simulink model "simulate_FM_Baseband"  (R2021a)
settings: Solver=VariableStepAuto  StartTime=0.0  StopTime=inf  RelTol=1e-3
InitFcn:
  | fs = 1e5;
  | Ts = 1/fs;
  | frameSize=1024;
  | freqDev = 250; % Hz / (volt sec)
libraries: commchan3 x1, commanabbnd3 x1, commrflib2 x1, dspsrcs4 x1, simulink x1
settings Model: Creator=Byung-Jun Jang  LastModifiedBy=user
settings SolverCC: AlgebraicLoopSolver=TrustRegion
settings DataIOCC: ReturnWorkspaceOutputs=off
settings DebuggingCC: SFMachineParentedDataDiag=warning  ArithmeticOperatorsInVariantConditions=warning
settings SFSimCC: SimUseLocalCustomCode=off  CustomCodeUndefinedFunction=UseInterfaceOnly
settings RTWCC: RTWUseLocalCustomCode=off
settings CodeAppCC: StateflowObjectComments=on

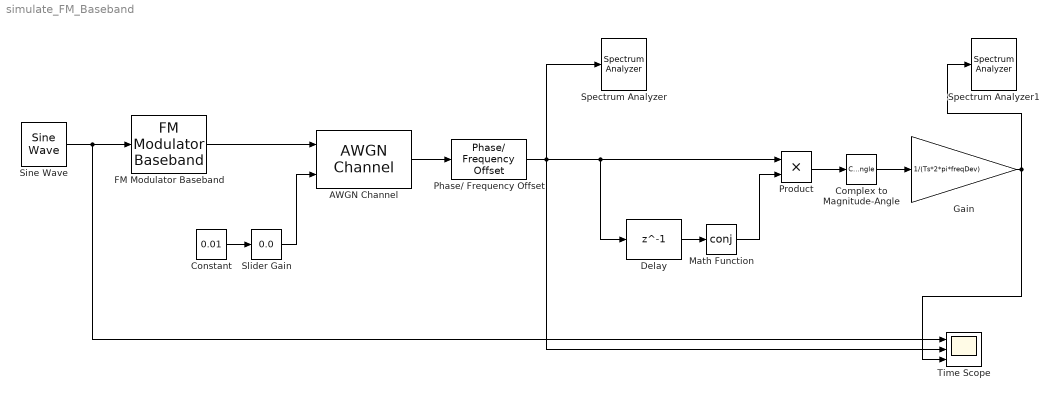
== system simulate_FM_Baseband ==
  AWGN Channel : commchan3/AWGN Channel  InputProcessing=Columns as channels (frame based)  seed=67  noiseMode=Variance from port  EbNodB=10  EsNodB=10  SNRdB=10  bitsPerSym=1  Ps=1  Tsym=1  variance=1
  Complex to Magnitude-Angle : ComplexToMagnitudeAngle  Output=Angle
  Constant : Constant  Value=0.01
  Delay : Delay  DelayLength=1  InputProcessing=Columns as channels (frame based)
  FM Modulator Baseband : commanabbnd3/FM Modulator Baseband  FrequencyDeviation=freqDev  SimulateUsing=Code generation
      settings: SourceProductBaseCode=CM
  Gain : Gain  Gain=1/(Ts*2*pi*freqDev)
  Math Function : Math  Operator=conj  SignedPower=on  SaturateOnIntegerOverflow=on
  Phase/ Frequency Offset : commrflib2/Phase// Frequency Offset  phaseOffset=180  freqPort=off  freqOffset=10
  Product : Product
  Sine Wave : dspsrcs4/Sine Wave  Amplitude=1  Frequency=1000  Phase=0  SampleMode=Discrete  OutComplex=Real  CompMethod=Trigonometric fcn  TableSize=Speed  SampleTime=Ts  SamplesPerFrame=frameSize  ResetState=Restart at time zero  OutputFrames=off  dataType=double  wordLen=16  udDataType=sfix(16)  fracBitsMode=Best precision  numFracBits=15  OutDataTypeStr=double  LastOutDataTypeStr=double
  Slider Gain : simulink/Math Operations/Slider Gain  gain=0.0  low=0  high=0.1
  Spectrum Analyzer : SpectrumAnalyzer
  Spectrum Analyzer1 : SpectrumAnalyzer
  Time Scope : Scope  NumInputPorts=3
  wires:
  Sine Wave/1 -> Time Scope/1, FM Modulator Baseband/1
  Delay/1 -> Math Function/1
  Complex to Magnitude-Angle/1 -> Gain/1
  FM Modulator Baseband/1 -> AWGN Channel/1
  Product/1 -> Complex to Magnitude-Angle/1
  Math Function/1 -> Product/2
  Gain/1 -> Spectrum Analyzer1/1, Time Scope/3
  Phase/ Frequency Offset/1 -> Time Scope/2, Spectrum Analyzer/1, Delay/1, Product/1
  AWGN Channel/1 -> Phase/ Frequency Offset/1
  Slider Gain/1 -> AWGN Channel/2
  Constant/1 -> Slider Gain/1
